simulink model "sim_1_2"  (R2022b)
settings: Solver=VariableStepAuto  StartTime=0.0  StopTime=20  FixedStep=0.001  MaxStep=0.001  RelTol=1e-3
values from neighbouring files (symbols this model uses):
  a_sin = [pi/2; pi/2; 0.2; pi/2]    [par_1_2.m]
  Kd = 30000*eye(4)    [par_1_2.m]
  Kp = 3000*eye(4)    [par_1_2.m]
  omega_sin = 10*[1; 1; 1; 1]    [par_1_2.m]
  q_0 = [0;0;0;0]    [par_1_2.m]
  q_dot_0 = [0;0;0;0]    [par_1_2.m]
undefined symbols (not defined in the file or in its folder): a_filt, b_filt
settings Model: Creator=Alberto  LastModifiedBy=david
settings SolverCC: AlgebraicLoopSolver=TrustRegion
settings DebuggingCC: UnconnectedInputMsg=warning  UnconnectedOutputMsg=warning  UnconnectedLineMsg=warning  SFMachineParentedDataDiag=warning
settings ModelReferenceCC: EnableRefExpFcnMdlSchedulingChecks=on
settings RTWCC: DLArmComputeVersion=19.05

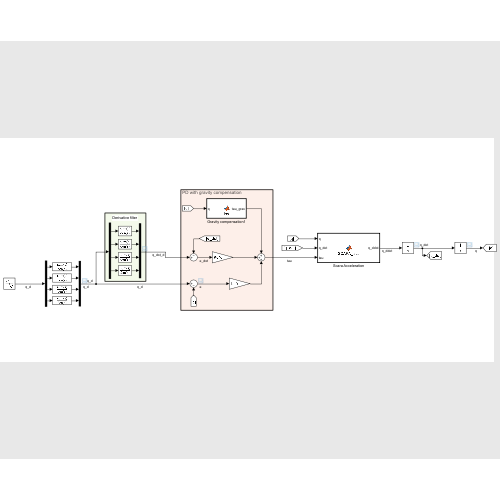
[thumbnail: Simulink's stored preview of the top-level diagram]
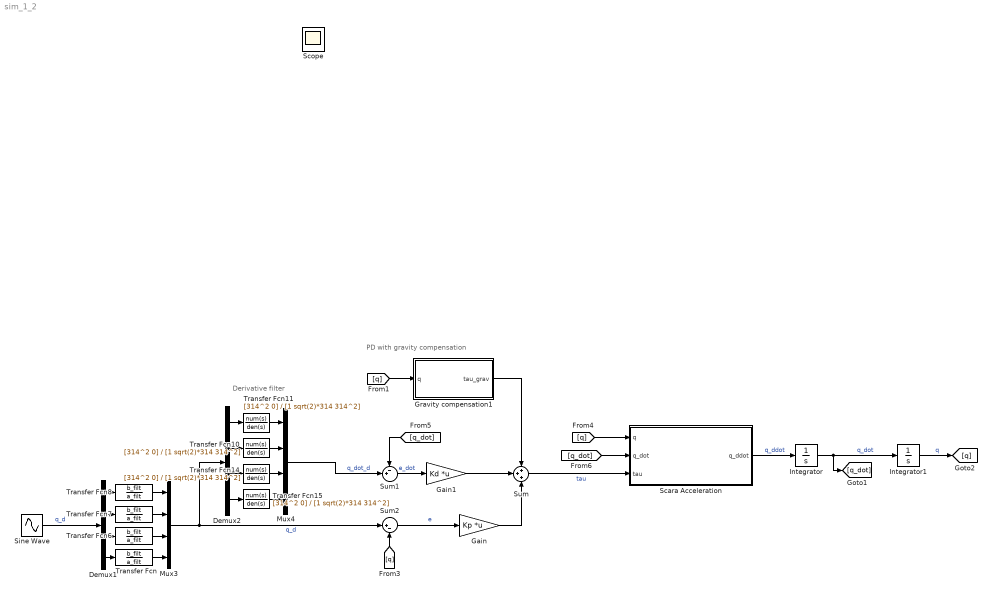
== system sim_1_2 ==
  note: PD with gravity compensation
  note: Derivative filter
  Demux1 : Demux
  Demux2 : Demux
  Gain : Gain  Gain=Kp  Multiplication=Matrix(K*u)
  Gain1 : Gain  Gain=Kd  Multiplication=Matrix(K*u)
  Gravity compensation1 : MATLAB Function  TreatAsAtomicUnit=on
  Integrator : Integrator  InitialCondition=q_dot_0
  Integrator1 : Integrator  InitialCondition=q_0
  Mux3 : Mux
  Mux4 : Mux
  Scara Acceleration : MATLAB Function  TreatAsAtomicUnit=on
  Sine Wave : Sin  Amplitude=a_sin  Frequency=omega_sin  SampleTime=0
  Sum : Sum  Inputs=+++
  Sum1 : Sum  Inputs=-+|
  Sum2 : Sum  Inputs=|+-
  Transfer Fcn{,6..8} (4 alike) : TransferFcn  Numerator=b_filt  Denominator=a_filt
  Transfer Fcn{10..11,14..15} (4 alike) : TransferFcn  Numerator=[314^2 0]  Denominator=[1 sqrt(2)*314 314^2]
  Scope : Scope
  wires:
  [q] -> Scara Acceleration/1(q)
  [q_dot] -> Sum1/1
  [q_dot] -> Scara Acceleration/2(q_dot)
  [q] -> Sum2/2
  Sum/1 -> Scara Acceleration/3(tau)  "tau"
  Scara Acceleration/1(q_ddot) -> Integrator/1  "q_ddot"
  Gain/1 -> Sum/3
  Sum1/1 -> Gain1/1  "e_dot"
  Integrator/1 -> [q_dot], Integrator1/1  "q_dot"
  Transfer Fcn/1 -> Mux3/4
  Gain1/1 -> Sum/2
  Transfer Fcn7/1 -> Mux3/2
  Transfer Fcn6/1 -> Mux3/3
  Demux1/2 -> Transfer Fcn7/1
  Demux1/3 -> Transfer Fcn6/1
  Integrator1/1 -> [q]  "q"
  Transfer Fcn8/1 -> Mux3/1
  Demux1/4 -> Transfer Fcn/1
  Sine Wave/1 -> Demux1/1  "q_d"
  Gravity compensation1/1(tau_grav) -> Sum/1
  [q] -> Gravity compensation1/1(q)
  Demux1/1 -> Transfer Fcn8/1
  Sum2/1 -> Gain/1  "e"
  Transfer Fcn11/1 -> Mux4/1
  Mux4/1 -> Sum1/2  "q_dot_d"
  Demux2/4 -> Transfer Fcn15/1
  Transfer Fcn14/1 -> Mux4/3
  Demux2/3 -> Transfer Fcn14/1
  Transfer Fcn10/1 -> Mux4/2
  Demux2/2 -> Transfer Fcn10/1
  Demux2/1 -> Transfer Fcn11/1
  Transfer Fcn15/1 -> Mux4/4
  Mux3/1 -> Demux2/1, Sum2/1  "q_d"

== matlab function sim_1_2/Scara Acceleration ==
  data: q input; q_ddot output; q_dot input; tau input
function q_ddot = SCARA_acc(q, q_dot, tau)%#codegen
coder.extrinsic('f_B_mex'); 
coder.extrinsic('f_C_vect_mex'); 
coder.extrinsic('f_g_vect_mex');
B = eye(4);
C_vect = zeros(4,1);
F_g = zeros(4,1);
tau = reshape(tau,4,1);
q_ddot = zeros(4,1);
B = full(f_B_mex('f_B',q));
C_vect = full(f_C_vect_mex('f_C_vect', q, q_dot));
F_g = full(f_g_vect_mex('f_g_vect', q));
q_ddot = (eye(4)/B)*(-C_vect-F_g+tau);

== matlab function sim_1_2/Gravity compensation1 ==
  data: q input; tau_grav output
function tau_grav = fcn(q)%#codegen
coder.extrinsic('f_g_vect_mex');
tau_grav = zeros(4,1);
tau_grav = reshape(full(f_g_vect_mex('f_g_vect', q)),4,1);
